simulink model "Block_Leg_PurePursuit"  (R2025b)
settings: Solver=VariableStepAuto  StartTime=0.0  StopTime=80  RelTol=1e-3  AbsTol=1e-3  EnableMultiTasking=on
undefined symbols (not defined in the file): waypoints, X, Y, Z
libraries: sm_lib x58, nesl_utility x34, slpidlib x2, robotalgslib x1, sharedtransform x1
(part 3 of 3)

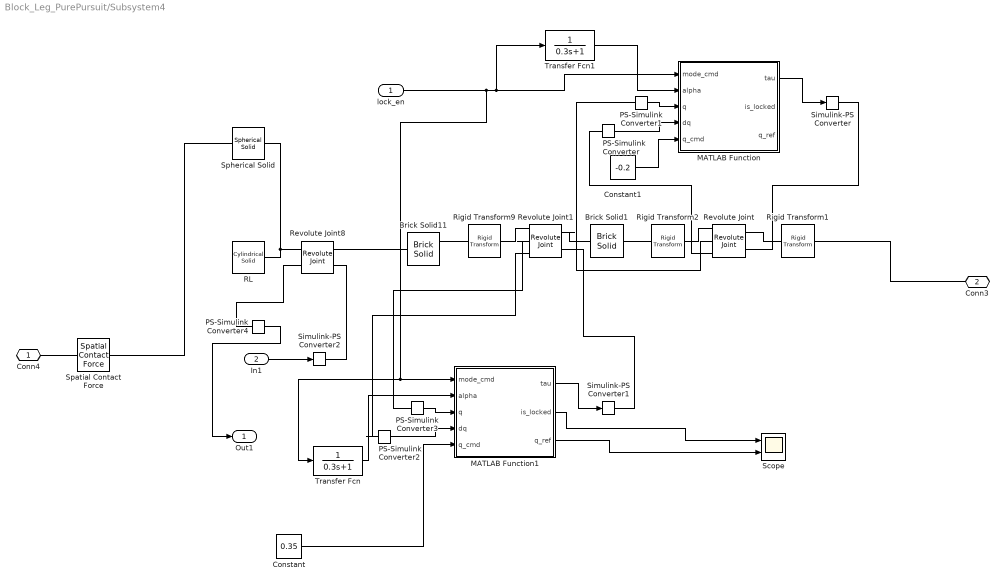
== system Block_Leg_PurePursuit/Subsystem4 ==
  lock_en : Inport
  In1 : Inport  Port=2
  Brick Solid1 : sm_lib/Body Elements/Brick Solid  BrickDimensions=[0.2 0.6 0.2]  BrickDimensionsUnits=m  ExportEntireGeometry=off  InertiaType=CalculateFromGeometry  BasedOnType=Mass  Density=1000  DensityUnits=kg/m^3  Mass=1  MassUnits=kg  CenterOfMass=[0 0 0]  CenterOfMassUnits=m  MomentsOfInertia=[1 1 1]  MomentsOfInertiaUnits=kg*m^2  ProductsOfInertia=[0 0 0]  ProductsOfInertiaUnits=kg*m^2  GraphicType=FromGeometry  MarkerShape=Sphere  MarkerSize=10  GraphicVisPropType=SimpleVisualProperties  GraphicDiffuseColor=[0.6667 1 1]  GraphicOpacity=1  GraphicSpecularColor=[0.5 0.5 0.5 1.0]  GraphicAmbientColor=[0.15 0.15 0.15 1.0]  GraphicEmissiveColor=[0.0 0.0 0.0 1.0]  GraphicShininess=75  DoExposeReferenceFrame=off  SerializedFrames=|
      | <Frames>
      | 
      |   <Frame>
      |     <Id>Frame1</Id>
      |     <Value>
      |       <Name>F1</Name>
      |       <Origin>
      |         <Source>GeometricFeature</Source>
      |         <FeatureName>+x -y +z point</FeatureName>
      |       </Origin>
      |       <PrimaryAxis>
      |         <DefinedDirection>+Z</DefinedDirection>
      |         <Source>ReferenceFrame</Source>
      |         <SourceDirection>+Z</SourceDirection>
      |         <FeatureName></FeatureName>
      |       </PrimaryAxis>
      |       <SecondaryAxis>
      |         <DefinedDirection>+X</DefinedDirection>
      |         <Source>ReferenceFrame</Source>
      |         <SourceDirection>+X</SourceDirection>
      |         <FeatureName></FeatureName>
      |       </SecondaryAxis>
      |     </Value>
      |   </Frame>
      | 
      |   <Frame>
      |     <Id>Frame2</Id>
      |     <Value>
      |       <Name>F2</Name>
      |       <Origin>
      |         <Source>GeometricFeature</Source>
      |         <FeatureName>+y surface</FeatureName>
      |       </Origin>
      |       <PrimaryAxis>
      |         <DefinedDirection>+Z</DefinedDirection>
      |         <Source>ReferenceFrame</Source>
      |         <SourceDirection>+Z</SourceDirection>
      |         <FeatureName></FeatureName>
      |       </PrimaryAxis>
      |       <SecondaryAxis>
      |         <DefinedDirection>+X</DefinedDirection>
      |         <Source>ReferenceFrame</Source>
      |         <SourceDirection>+X</SourceDirection>
      |         <FeatureName></FeatureName>
      |       </SecondaryAxis>
      |     </Value>
      |   </Frame>
      | 
      | </Frames>
  Brick Solid11 : sm_lib/Body Elements/Brick Solid  BrickDimensions=[0.2 1 0.2]  BrickDimensionsUnits=m  ExportEntireGeometry=on  InertiaType=CalculateFromGeometry  BasedOnType=Mass  Density=1000  DensityUnits=kg/m^3  Mass=1  MassUnits=kg  CenterOfMass=[0 0 0]  CenterOfMassUnits=m  MomentsOfInertia=[1 1 1]  MomentsOfInertiaUnits=kg*m^2  ProductsOfInertia=[0 0 0]  ProductsOfInertiaUnits=kg*m^2  GraphicType=FromGeometry  MarkerShape=Sphere  MarkerSize=10  GraphicVisPropType=SimpleVisualProperties  GraphicDiffuseColor=[0.6667 1 1]  GraphicOpacity=1  GraphicSpecularColor=[0.5 0.5 0.5 1.0]  GraphicAmbientColor=[0.15 0.15 0.15 1.0]  GraphicEmissiveColor=[0.0 0.0 0.0 1.0]  GraphicShininess=75  DoExposeReferenceFrame=off  SerializedFrames=|
      | <Frames>
      | 
      |   <Frame>
      |     <Id>Frame1</Id>
      |     <Value>
      |       <Name>F1</Name>
      |       <Origin>
      |         <Source>GeometricFeature</Source>
      |         <FeatureName>+x -y +z point</FeatureName>
      |       </Origin>
      |       <PrimaryAxis>
      |         <DefinedDirection>+Z</DefinedDirection>
      |         <Source>ReferenceFrame</Source>
      |         <SourceDirection>+Z</SourceDirection>
      |         <FeatureName></FeatureName>
      |       </PrimaryAxis>
      |       <SecondaryAxis>
      |         <DefinedDirection>+X</DefinedDirection>
      |         <Source>ReferenceFrame</Source>
      |         <SourceDirection>+X</SourceDirection>
      |         <FeatureName></FeatureName>
      |       </SecondaryAxis>
      |     </Value>
      |   </Frame>
      | 
      |   <Frame>
      |     <Id>Frame2</Id>
      |     <Value>
      |       <Name>F2</Name>
      |       <Origin>
      |         <Source>GeometricFeature</Source>
      |         <FeatureName>+y surface</FeatureName>
      |       </Origin>
      |       <PrimaryAxis>
      |         <DefinedDirection>+Z</DefinedDirection>
      |         <Source>ReferenceFrame</Source>
      |         <SourceDirection>+Z</SourceDirection>
      |         <FeatureName></FeatureName>
      |       </PrimaryAxis>
      |       <SecondaryAxis>
      |         <DefinedDirection>+X</DefinedDirection>
      |         <Source>ReferenceFrame</Source>
      |         <SourceDirection>+X</SourceDirection>
      |         <FeatureName></FeatureName>
      |       </SecondaryAxis>
      |     </Value>
      |   </Frame>
      | 
      | </Frames>
  Constant : Constant  Value=0.35
  Constant1 : Constant  Value=-0.2
  MATLAB Function : MATLAB Function  TreatAsAtomicUnit=on  SystemSampleTime=0.002
  MATLAB Function1 : MATLAB Function  TreatAsAtomicUnit=on  SystemSampleTime=0.002
  PS-Simulink Converter{,1..4} (5 alike) : nesl_utility/PS-Simulink Converter  PhysicalDomain=network_engine_domain  SubClassName=ps_output  LeftPortType=input  RightPortType=output  PseudoPeriodic=off  Frequencies=[]  VectorFormat=inherit  Unit=inherit  AffineConversion=off
  RL : sm_lib/Body Elements/Cylindrical Solid  CylinderRadius=0.5  CylinderRadiusUnits=m  CylinderLength=0.3  CylinderLengthUnits=m  ExportEntireGeometry=on  InertiaType=CalculateFromGeometry  BasedOnType=Mass  Density=1000  DensityUnits=kg/m^3  Mass=0.2  MassUnits=kg  CenterOfMass=[0 0 0]  CenterOfMassUnits=m  MomentsOfInertia=[1 1 1]  MomentsOfInertiaUnits=kg*m^2  ProductsOfInertia=[0 0 0]  ProductsOfInertiaUnits=kg*m^2  GraphicType=FromGeometry  MarkerShape=Sphere  MarkerSize=10  GraphicVisPropType=SimpleVisualProperties  GraphicDiffuseColor=[0.6667 1 1]  GraphicOpacity=1  GraphicSpecularColor=[0.5 0.5 0.5 1.0]  GraphicAmbientColor=[0.15 0.15 0.15 1.0]  GraphicEmissiveColor=[0.0 0.0 0.0 1.0]  GraphicShininess=75  DoExposeReferenceFrame=on  SerializedFrames=<Frames/>
  Revolute Joint : sm_lib/Joints/Revolute Joint  JointMode=Normal  CompositeWrenchDir=FollowerOnBase  CompositeWrenchFrame=BaseFrame  SenseConstraintForce=off  SenseConstraintTorque=off  SenseTotalForce=off  SenseTotalTorque=off  PositionTargetSpecify=off  PositionTargetPriority=High  PositionTargetValue=0  PositionTargetValueUnits=deg  VelocityTargetSpecify=off  VelocityTargetPriority=High  VelocityTargetValue=0  VelocityTargetValueUnits=deg/s  EquilibriumPosition=0  EquilibriumPositionUnits=deg  SpringStiffness=0  SpringStiffnessUnits=N*m/deg  DampingCoefficient=0  DampingCoefficientUnits=N*m/(deg/s)  LowerLimitSpecify=off  LowerLimitBound=-90  LowerLimitBoundUnits=deg  LowerLimitStiffness=1e4  LowerLimitStiffnessUnits=N*m/deg  LowerLimitDamping=10  LowerLimitDampingUnits=N*m/(deg/s)  LowerLimitTransitionRegionWidth=0.1  LowerLimitTransitionRegionWidthUnits=deg  UpperLimitSpecify=off  UpperLimitBound=90  UpperLimitBoundUnits=deg  UpperLimitStiffness=1e4  UpperLimitStiffnessUnits=N*m/deg  UpperLimitDamping=10  UpperLimitDampingUnits=N*m/(deg/s)  UpperLimitTransitionRegionWidth=0.1  UpperLimitTransitionRegionWidthUnits=deg  TorqueActuationMode=InputTorque  MotionActuationMode=ComputedMotion  SensePosition=on  SenseVelocity=on  SenseAcceleration=off  SenseTorqueForce=off  SenseLowerLimitTorqueForce=off  SenseUpperLimitTorqueForce=off
  Revolute Joint1 : sm_lib/Joints/Revolute Joint  JointMode=Normal  CompositeWrenchDir=FollowerOnBase  CompositeWrenchFrame=BaseFrame  SenseConstraintForce=off  SenseConstraintTorque=off  SenseTotalForce=off  SenseTotalTorque=off  PositionTargetSpecify=off  PositionTargetPriority=High  PositionTargetValue=0  PositionTargetValueUnits=deg  VelocityTargetSpecify=off  VelocityTargetPriority=High  VelocityTargetValue=0  VelocityTargetValueUnits=deg/s  EquilibriumPosition=0  EquilibriumPositionUnits=deg  SpringStiffness=0  SpringStiffnessUnits=N*m/deg  DampingCoefficient=0  DampingCoefficientUnits=N*m/(deg/s)  LowerLimitSpecify=off  LowerLimitBound=-90  LowerLimitBoundUnits=deg  LowerLimitStiffness=1e4  LowerLimitStiffnessUnits=N*m/deg  LowerLimitDamping=10  LowerLimitDampingUnits=N*m/(deg/s)  LowerLimitTransitionRegionWidth=0.1  LowerLimitTransitionRegionWidthUnits=deg  UpperLimitSpecify=off  UpperLimitBound=90  UpperLimitBoundUnits=deg  UpperLimitStiffness=1e4  UpperLimitStiffnessUnits=N*m/deg  UpperLimitDamping=10  UpperLimitDampingUnits=N*m/(deg/s)  UpperLimitTransitionRegionWidth=0.1  UpperLimitTransitionRegionWidthUnits=deg  TorqueActuationMode=InputTorque  MotionActuationMode=ComputedMotion  SensePosition=on  SenseVelocity=on  SenseAcceleration=off  SenseTorqueForce=off  SenseLowerLimitTorqueForce=off  SenseUpperLimitTorqueForce=off
  Revolute Joint8 : sm_lib/Joints/Revolute Joint  JointMode=Normal  CompositeWrenchDir=FollowerOnBase  CompositeWrenchFrame=BaseFrame  SenseConstraintForce=off  SenseConstraintTorque=off  SenseTotalForce=off  SenseTotalTorque=off  PositionTargetSpecify=off  PositionTargetPriority=High  PositionTargetValue=0  PositionTargetValueUnits=deg  VelocityTargetSpecify=off  VelocityTargetPriority=High  VelocityTargetValue=0  VelocityTargetValueUnits=deg/s  EquilibriumPosition=0  EquilibriumPositionUnits=deg  SpringStiffness=0  SpringStiffnessUnits=N*m/deg  DampingCoefficient=0  DampingCoefficientUnits=N*m/(deg/s)  LowerLimitSpecify=off  LowerLimitBound=-90  LowerLimitBoundUnits=deg  LowerLimitStiffness=1e4  LowerLimitStiffnessUnits=N*m/deg  LowerLimitDamping=10  LowerLimitDampingUnits=N*m/(deg/s)  LowerLimitTransitionRegionWidth=0.1  LowerLimitTransitionRegionWidthUnits=deg  UpperLimitSpecify=off  UpperLimitBound=90  UpperLimitBoundUnits=deg  UpperLimitStiffness=1e4  UpperLimitStiffnessUnits=N*m/deg  UpperLimitDamping=10  UpperLimitDampingUnits=N*m/(deg/s)  UpperLimitTransitionRegionWidth=0.1  UpperLimitTransitionRegionWidthUnits=deg  TorqueActuationMode=InputTorque  MotionActuationMode=ComputedMotion  SensePosition=off  SenseVelocity=on  SenseAcceleration=off  SenseTorqueForce=off  SenseLowerLimitTorqueForce=off  SenseUpperLimitTorqueForce=off
  Rigid Transform1 : sm_lib/Frames and Transforms/Rigid Transform  RotationMethod=AlignedAxes  FollAlignAxisA=+Z  BaseAlignAxisA=+Y  FollAlignAxisB=+X  BaseAlignAxisB=+X  RotationStandardAxis=+Z  RotationAngle=0  RotationAngleUnits=deg  RotationArbitraryAxis=[0 0 1]  RotationSequenceAxes=FollowerAxes  RotationSequence=XYX  RotationSequenceAngles=[0 0 0]  RotationSequenceAnglesUnits=deg  RotationMatrix=[1 0 0;0 1 0;0 0 1]  Quaternion=[1 0 0 0]  TranslationMethod=None  TranslationCartesianOffset=[0 0 0]  TranslationCartesianOffsetUnits=m  TranslationStandardAxis=+Z  TranslationStandardOffset=0  TranslationStandardOffsetUnits=m  TranslationROffset=0  TranslationROffsetUnits=m  TranslationThetaOffset=0  TranslationThetaOffsetUnits=deg  TranslationZOffset=0  TranslationZOffsetUnits=m
  Rigid Transform2 : sm_lib/Frames and Transforms/Rigid Transform  RotationMethod=RotationSequence  FollAlignAxisA=+X  BaseAlignAxisA=+Y  FollAlignAxisB=+Y  BaseAlignAxisB=+Z  RotationStandardAxis=+Z  RotationAngle=0  RotationAngleUnits=deg  RotationArbitraryAxis=[0 0 1]  RotationSequenceAxes=FollowerAxes  RotationSequence=XYZ  RotationSequenceAngles=[0 0 45]  RotationSequenceAnglesUnits=deg  RotationMatrix=[1 0 0;0 1 0;0 0 1]  Quaternion=[1 0 0 0]  TranslationMethod=None  TranslationCartesianOffset=[0 0 0]  TranslationCartesianOffsetUnits=m  TranslationStandardAxis=+Z  TranslationStandardOffset=0  TranslationStandardOffsetUnits=m  TranslationROffset=0  TranslationROffsetUnits=m  TranslationThetaOffset=0  TranslationThetaOffsetUnits=deg  TranslationZOffset=0  TranslationZOffsetUnits=m
  Rigid Transform9 : sm_lib/Frames and Transforms/Rigid Transform  RotationMethod=RotationSequence  FollAlignAxisA=+X  BaseAlignAxisA=+Y  FollAlignAxisB=+Y  BaseAlignAxisB=+Z  RotationStandardAxis=+Z  RotationAngle=0  RotationAngleUnits=deg  RotationArbitraryAxis=[0 0 1]  RotationSequenceAxes=FollowerAxes  RotationSequence=XYZ  RotationSequenceAngles=[0 0 -75]  RotationSequenceAnglesUnits=deg  RotationMatrix=[1 0 0;0 1 0;0 0 1]  Quaternion=[1 0 0 0]  TranslationMethod=None  TranslationCartesianOffset=[0 0 0]  TranslationCartesianOffsetUnits=m  TranslationStandardAxis=+Z  TranslationStandardOffset=0  TranslationStandardOffsetUnits=m  TranslationROffset=0  TranslationROffsetUnits=m  TranslationThetaOffset=0  TranslationThetaOffsetUnits=deg  TranslationZOffset=0  TranslationZOffsetUnits=m
  Scope : Scope  NumInputPorts=2
      settings: ActiveDisplayYMinimum=-1  ActiveDisplayYMaximum=1
  Simulink-PS Converter : nesl_utility/Simulink-PS Converter  PhysicalDomain=network_engine_domain  SubClassName=ps_input  LeftPortType=input  RightPortType=output  PseudoPeriodic=off  Frequencies=[]  NoiseDistribution=none  NoiseParameters=[]  Unit=1  AffineConversion=off  FilteringAndDerivatives=provide  SimscapeFilterOrder=1  InputFilterTimeConstant=0.001  UdotUserProvided=0
  Simulink-PS Converter1 : nesl_utility/Simulink-PS Converter  PhysicalDomain=network_engine_domain  SubClassName=ps_input  LeftPortType=input  RightPortType=output  PseudoPeriodic=off  Frequencies=[]  NoiseDistribution=none  NoiseParameters=[]  Unit=1  AffineConversion=off  FilteringAndDerivatives=provide  SimscapeFilterOrder=1  InputFilterTimeConstant=0.001  UdotUserProvided=0
  Simulink-PS Converter2 : nesl_utility/Simulink-PS Converter  PhysicalDomain=network_engine_domain  SubClassName=ps_input  LeftPortType=input  RightPortType=output  PseudoPeriodic=off  Frequencies=[]  NoiseDistribution=none  NoiseParameters=[]  Unit=1  AffineConversion=off  FilteringAndDerivatives=provide  SimscapeFilterOrder=1  InputFilterTimeConstant=0.001  UdotUserProvided=0
  Spatial Contact Force : sm_lib/Forces and Torques/Spatial Contact Force  SenseSeparationDistance=off  NormalForceType=SmoothSpringDamper  NormalStiffness=1e6  NormalStiffnessUnits=N/m  NormalDamping=1e3  NormalDampingUnits=N/(m/s)  NormalTransitionRegionWidth=1e-4  NormalTransitionRegionWidthUnits=m  FrictionType=SmoothStickSlip  CoefficientOfStaticFriction=0.9  CoefficientOfDynamicFriction=0.7  FrictionalCriticalVelocity=1e-3  FrictionalCriticalVelocityUnits=m/s  SenseContactSignal=off  SensePenetrationDepth=off  SenseNormalVelocity=off  SenseTangentialVelocity=off  SensingForceTorqueDirection=BaseOnFollower  SensingForceTorqueResolutionFrame=ContactFrame  SenseNormalForce=off  SenseNormalForceMagnitude=off  SenseNormalTorque=off  SenseFrictionalForce=off  SenseFrictionalForceMagnitude=off  SenseFrictionalTorque=off  SenseTotalForce=off  SenseTotalTorque=off  SenseContactBaseRotation=off  SenseContactBaseTranslation=off  SenseContactFollowerRotation=off  SenseContactFollowerTranslation=off  ZeroCrossDetectContactStartAndEnd=off
  Spherical Solid : sm_lib/Body Elements/Spherical Solid  SphereRadius=0.5  SphereRadiusUnits=m  ExportEntireGeometry=on  InertiaType=CalculateFromGeometry  BasedOnType=Mass  Density=1000  DensityUnits=kg/m^3  Mass=0  MassUnits=kg  CenterOfMass=[0 0 0]  CenterOfMassUnits=m  MomentsOfInertia=[1 1 1]  MomentsOfInertiaUnits=kg*m^2  ProductsOfInertia=[0 0 0]  ProductsOfInertiaUnits=kg*m^2  GraphicType=FromGeometry  MarkerShape=Sphere  MarkerSize=10  GraphicVisPropType=SimpleVisualProperties  GraphicDiffuseColor=[1 0 0]  GraphicOpacity=0.2  GraphicSpecularColor=[0.5 0.5 0.5 1.0]  GraphicAmbientColor=[0.15 0.15 0.15 1.0]  GraphicEmissiveColor=[0.0 0.0 0.0 1.0]  GraphicShininess=75  DoExposeReferenceFrame=on  SerializedFrames=<Frames/>
  Transfer Fcn : TransferFcn  Denominator=[0.3 1]
  Transfer Fcn1 : TransferFcn  Denominator=[0.3 1]
  Conn4 : PMIOPort  Side=Left
  Conn3 : PMIOPort  Port=2  Side=Right
  Out1 : Outport
  wires:
  MATLAB Function/1(tau) -> Simulink-PS Converter/1
  PS-Simulink Converter3/1 -> MATLAB Function1/3(q)
  PS-Simulink Converter2/1 -> MATLAB Function1/4(dq)
  PS-Simulink Converter/1 -> MATLAB Function/4(dq)
  PS-Simulink Converter1/1 -> MATLAB Function/3(q)
  MATLAB Function1/1(tau) -> Simulink-PS Converter1/1
  In1/1 -> Simulink-PS Converter2/1
  PS-Simulink Converter4/1 -> Out1/1
  MATLAB Function1/2(is_locked) -> Scope/1
  MATLAB Function1/3(q_ref) -> Scope/2
  Transfer Fcn/1 -> MATLAB Function1/2(alpha)
  Transfer Fcn1/1 -> MATLAB Function/2(alpha)
  lock_en/1 -> Transfer Fcn/1, MATLAB Function1/1(mode_cmd), Transfer Fcn1/1, MATLAB Function/1(mode_cmd)
  Constant/1 -> MATLAB Function1/5(q_cmd)
  Constant1/1 -> MATLAB Function/5(q_cmd)
  connections:
  Revolute Joint/LConn1 -- Rigid Transform1/RConn1
  Simulink-PS Converter1/RConn1 -- Revolute Joint1/LConn2
  Rigid Transform9/LConn1 -- Revolute Joint1/RConn1
  Spherical Solid/LConn1 -- Spatial Contact Force/RConn1
  Brick Solid11/RConn1 -- Revolute Joint8/LConn1
  Revolute Joint1/LConn1 -- Brick Solid1/RConn1
  Revolute Joint8/RConn1 -- RL/RConn1 -- Spherical Solid/RConn1
  Rigid Transform2/LConn1 -- Revolute Joint/RConn1
  Brick Solid11/LConn1 -- Rigid Transform9/RConn1
  Brick Solid1/LConn1 -- Rigid Transform2/RConn1
  Spatial Contact Force/LConn1 -- Conn4/RConn1
  PS-Simulink Converter2/LConn1 -- Revolute Joint1/RConn3
  PS-Simulink Converter/LConn1 -- Revolute Joint/RConn3
  Revolute Joint1/RConn2 -- PS-Simulink Converter3/LConn1
  Simulink-PS Converter/RConn1 -- Revolute Joint/LConn2
  PS-Simulink Converter1/LConn1 -- Revolute Joint/RConn2
  Rigid Transform1/LConn1 -- Conn3/RConn1
  Simulink-PS Converter2/RConn1 -- Revolute Joint8/LConn2
  Revolute Joint8/RConn2 -- PS-Simulink Converter4/LConn1

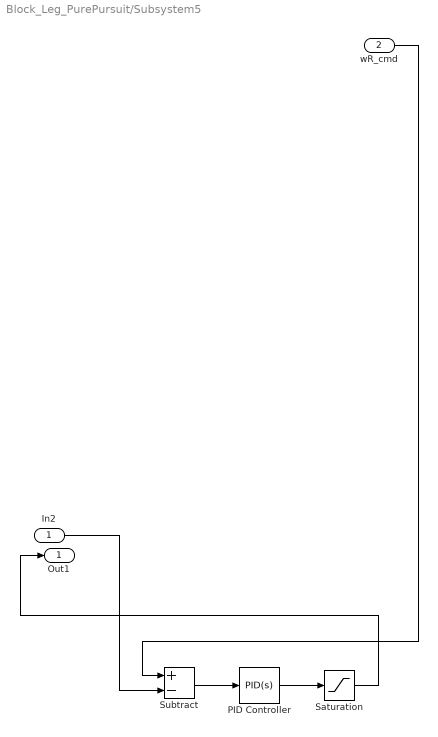
== system Block_Leg_PurePursuit/Subsystem5 ==
  In2 : Inport
  wR_cmd : Inport  Port=2
  PID Controller : slpidlib/PID Controller  Controller=PID  Form=Parallel  TimeDomain=Continuous-time  UseExternalTs=off  SampleTime=-1  IntegratorMethod=Forward Euler  FilterMethod=Forward Euler  ControllerParametersSource=internal  P=5  I=0  UseKiTs=off  D=0  UseExternalDerivativeSource=off  N=100  UseFilter=on  TunerSelectOption=Transfer Function Based (PID Tuner App)  InitialConditionSource=internal  InitialConditionForIntegrator=0  InitialConditionForFilter=0  DifferentiatorICPrevScaledInput=0  ExternalReset=none  TrackingMode=off  Kt=1  LimitOutput=off  SatLimitsSource=internal  UpperSaturationLimit=inf  LowerSaturationLimit=-inf  LinearizeAsGain=on  AntiWindupMode=none  Kb=1  LimitIntegrator=off  UpperIntegratorSaturationLimit=inf  LowerIntegratorSaturationLimit=-inf  POutMin=[]  POutMax=[]  IOutMin=[]  IOutMax=[]  DOutMin=[]  DOutMax=[]  NOutMin=[]  NOutMax=[]  SumOutMin=[]  SumOutMax=[]  SaturationOutMin=[]  SaturationOutMax=[]  PParamMin=[]  PParamMax=[]  IParamMin=[]  IParamMax=[]  DParamMin=[]  DParamMax=[]  NParamMin=[]  NParamMax=[]  KbParamMin=[]  KbParamMax=[]  KtParamMin=[]  KtParamMax=[]  KbOutMin=[]  KbOutMax=[]  KtOutMin=[]  KtOutMax=[]  IntegratorOutMin=[]  IntegratorOutMax=[]  FilterOutMin=[]  FilterOutMax=[]  SumI1OutMin=[]  SumI1OutMax=[]  SumI2OutMin=[]  SumI2OutMax=[]  SumI3OutMin=[]  SumI3OutMax=[]  SumI4OutMin=[]  SumI4OutMax=[]  SumDOutMin=[]  SumDOutMax=[]  DifferentiatorOutMin=[]  DifferentiatorOutMax=[]  FilterDiffOutCoefMin=[]  FilterDiffOutCoefMax=[]  ReciprocalOutMin=[]  ReciprocalOutMax=[]  SumDenOutMin=[]  SumDenOutMax=[]  SumNumOutMin=[]  SumNumOutMax=[]  DivideOutMin=[]  DivideOutMax=[]  UdiffTsProdOutMin=[]  UdiffTsProdOutMax=[]  NTsProdOutMin=[]  NTsProdOutMax=[]  UintegralTsProdOutMin=[]  UintegralTsProdOutMax=[]  UngainTsProdOutMin=[]  UngainTsProdOutMax=[]  ClampingZeroOutDataTypeStr=Inherit: Inherit via back propagation  ClampingZeroOutMin=[]  ClampingZeroOutMax=[]  FilterDenConstantOutDataTypeStr=Inherit: Inherit via back propagation  FilterDenConstantOutMin=[]  FilterDenConstantOutMax=[]  PCopyOutDataTypeStr=Inherit: Inherit via back propagation  PCopyOutMin=[]  PCopyOutMax=[]  NCopyOutDataTypeStr=Inherit: Inherit via back propagation  NCopyOutMin=[]  NCopyOutMax=[]  IntegratorContinuousStateAttributes=''  IntegratorStateMustResolveToSignalObject=off  IntegratorRTWStateStorageClass=Auto  FilterContinuousStateAttributes=''  FilterStateMustResolveToSignalObject=off  FilterRTWStateStorageClass=Auto  ParallelPVariant=InternalParameters  IdealPVariant=Disabled  IVariant=InternalParameters  DVariant=InternalParameters  IntegratorVariant=Continuous  SatVariant=Disabled  AWVariant=Passthrough  PCopyVariant=Disabled  TRVariant=Disabled  FdbkBlocksVariant=Forward  IdealPFdbkVariant=Disabled  SatFdbkVariant=Disabled  DerivativeFilterVariant=ContFilter  NVariant=InternalParameters  NCopyVariant=Disabled  FilterICVariant=InternalICsFilter  IntegratorICVariant=InternalICs  ExternalResetVariant=Disabled  TRSumVariant=Passthrough  SumFdbkVariant=Disabled  SumVariant=Sum_PID  TsampFilterVariant=InternalTs  TsampNgainVariant=Passthrough  TsampIntegralVariant=Disabled_SignalSpec  ExternalSaturationOutDataTypeStr=Inherit: Same as second input  DerivativeSourceVariant=ErrorSignal  PreIntVariant=InternalPreInt
  Saturation : Saturate  UpperLimit=5  LowerLimit=-5
  Subtract : Sum  Inputs=+-
  Out1 : Outport
  wires:
  In2/1 -> Subtract/2
  Subtract/1 -> PID Controller/1
  Saturation/1 -> Out1/1
  PID Controller/1 -> Saturation/1
  wR_cmd/1 -> Subtract/1

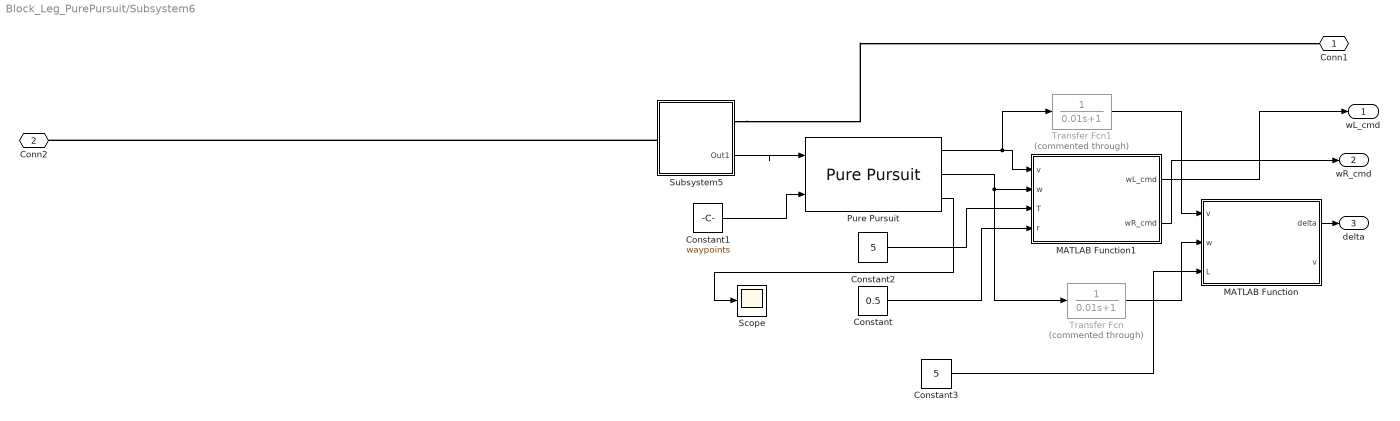
== system Block_Leg_PurePursuit/Subsystem6 ==
  Constant : Constant  Value=0.5
  Constant1 : Constant  Value=waypoints
  Constant2 : Constant  Value=5
  Constant3 : Constant  Value=5
  MATLAB Function : MATLAB Function  TreatAsAtomicUnit=on
  MATLAB Function1 : MATLAB Function  TreatAsAtomicUnit=on
  Pure Pursuit : robotalgslib/Pure Pursuit  DesiredLinearVelocityPort=off  DesiredLinearVelocity=3  MaxAngularVelocity=2  LookaheadDistancePort=off  LookaheadDistance=4  TargetDirPort=on  SimulateUsing=Code generation
      settings: LibrarySourceBlock=navlib/Control Algorithms/Pure Pursuit
  Scope : Scope
      settings: ActiveDisplayYMinimum=-4.8040636325719674  ActiveDisplayYMaximum=3.5962705540777251
  Subsystem5 : Subsystem
      settings: PortSchema="{\"entries\":[{\"content\":{\"sides\":[{\"content\":{\"connectorIds\":[\"LConn1\"]},\"type\":\"ConnectorPlacement.EquallySpacedRectSide\",\"uuid\":\"ddf93349-53d1-49a0-944e-d0734f46f29a\"},{\"content\":{\"connectorIds\":[\"RConn1\",\"Out1\"],\"side\":\"RIGHT\"},\"type\":\"ConnectorPlacement.EquallySpacedRectSide\",\"uuid\":\"41423d35-5168-4258-b195-077866701bba\"},{\"content\":{\"side\":\"TOP\"},\"type\":\"ConnectorPlacement.EquallySpacedRectSide\",\"uuid\":\"a64c51dc-c679-4f29-97b2-168705ea0e49\"}]},\"type\":\"ConnectorPlacement.EquallySpacedConnector\",\"uuid\":\"ed4aabc3-31ac-4b26-a964-31268bbe4985\"}],\"packageUris\":[\"http://schema.mathworks.com/mf0/Connector/R2020b\"],\"version\":\"1.0\"}"
  Transfer Fcn : TransferFcn  Commented=through  Denominator=[0.01 1]
  Transfer Fcn1 : TransferFcn  Commented=through  Denominator=[0.01 1]
  Conn1 : PMIOPort  Side=Right
  Conn2 : PMIOPort  Port=2  Side=Left
  wL_cmd : Outport
  wR_cmd : Outport  Port=2
  delta : Outport  Port=3
  wires:
  Pure Pursuit/2 -> Transfer Fcn/1, MATLAB Function1/2(w)
  Transfer Fcn1/1 -> MATLAB Function/1("v ")
  Transfer Fcn/1 -> MATLAB Function/2(w)
  Constant1/1 -> Pure Pursuit/2
  MATLAB Function/1(delta) -> delta/1
  Constant/1 -> MATLAB Function1/4(r)
  Constant2/1 -> MATLAB Function1/3(T)
  Constant3/1 -> MATLAB Function/3(L)
  MATLAB Function1/2(wR_cmd) -> wR_cmd/1
  MATLAB Function1/1(wL_cmd) -> wL_cmd/1
  Pure Pursuit/1 -> Transfer Fcn1/1, MATLAB Function1/1(v)
  Pure Pursuit/3 -> Scope/1
  Subsystem5/1(Out1) -> Pure Pursuit/1
  connections:
  Subsystem5/RConn1 -- Conn1/RConn1
  Subsystem5/LConn1 -- Conn2/RConn1

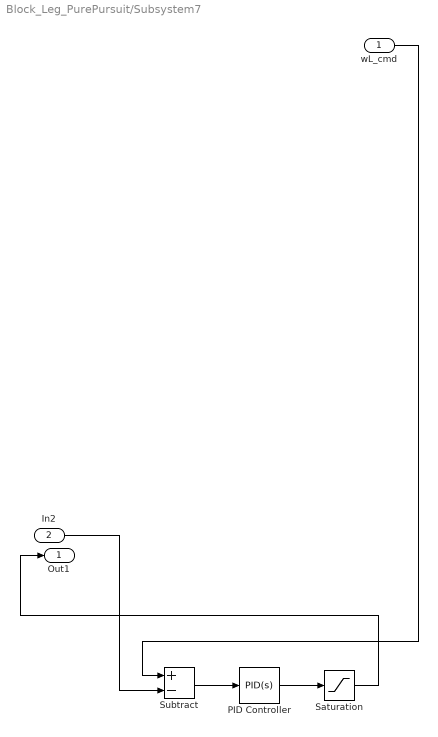
== system Block_Leg_PurePursuit/Subsystem7 ==
  wL_cmd : Inport
  In2 : Inport  Port=2
  PID Controller : slpidlib/PID Controller  Controller=PID  Form=Parallel  TimeDomain=Continuous-time  UseExternalTs=off  SampleTime=-1  IntegratorMethod=Forward Euler  FilterMethod=Forward Euler  ControllerParametersSource=internal  P=5  I=0  UseKiTs=off  D=0  UseExternalDerivativeSource=off  N=100  UseFilter=on  TunerSelectOption=Transfer Function Based (PID Tuner App)  InitialConditionSource=internal  InitialConditionForIntegrator=0  InitialConditionForFilter=0  DifferentiatorICPrevScaledInput=0  ExternalReset=none  TrackingMode=off  Kt=1  LimitOutput=off  SatLimitsSource=internal  UpperSaturationLimit=inf  LowerSaturationLimit=-inf  LinearizeAsGain=on  AntiWindupMode=none  Kb=1  LimitIntegrator=off  UpperIntegratorSaturationLimit=inf  LowerIntegratorSaturationLimit=-inf  POutMin=[]  POutMax=[]  IOutMin=[]  IOutMax=[]  DOutMin=[]  DOutMax=[]  NOutMin=[]  NOutMax=[]  SumOutMin=[]  SumOutMax=[]  SaturationOutMin=[]  SaturationOutMax=[]  PParamMin=[]  PParamMax=[]  IParamMin=[]  IParamMax=[]  DParamMin=[]  DParamMax=[]  NParamMin=[]  NParamMax=[]  KbParamMin=[]  KbParamMax=[]  KtParamMin=[]  KtParamMax=[]  KbOutMin=[]  KbOutMax=[]  KtOutMin=[]  KtOutMax=[]  IntegratorOutMin=[]  IntegratorOutMax=[]  FilterOutMin=[]  FilterOutMax=[]  SumI1OutMin=[]  SumI1OutMax=[]  SumI2OutMin=[]  SumI2OutMax=[]  SumI3OutMin=[]  SumI3OutMax=[]  SumI4OutMin=[]  SumI4OutMax=[]  SumDOutMin=[]  SumDOutMax=[]  DifferentiatorOutMin=[]  DifferentiatorOutMax=[]  FilterDiffOutCoefMin=[]  FilterDiffOutCoefMax=[]  ReciprocalOutMin=[]  ReciprocalOutMax=[]  SumDenOutMin=[]  SumDenOutMax=[]  SumNumOutMin=[]  SumNumOutMax=[]  DivideOutMin=[]  DivideOutMax=[]  UdiffTsProdOutMin=[]  UdiffTsProdOutMax=[]  NTsProdOutMin=[]  NTsProdOutMax=[]  UintegralTsProdOutMin=[]  UintegralTsProdOutMax=[]  UngainTsProdOutMin=[]  UngainTsProdOutMax=[]  ClampingZeroOutDataTypeStr=Inherit: Inherit via back propagation  ClampingZeroOutMin=[]  ClampingZeroOutMax=[]  FilterDenConstantOutDataTypeStr=Inherit: Inherit via back propagation  FilterDenConstantOutMin=[]  FilterDenConstantOutMax=[]  PCopyOutDataTypeStr=Inherit: Inherit via back propagation  PCopyOutMin=[]  PCopyOutMax=[]  NCopyOutDataTypeStr=Inherit: Inherit via back propagation  NCopyOutMin=[]  NCopyOutMax=[]  IntegratorContinuousStateAttributes=''  IntegratorStateMustResolveToSignalObject=off  IntegratorRTWStateStorageClass=Auto  FilterContinuousStateAttributes=''  FilterStateMustResolveToSignalObject=off  FilterRTWStateStorageClass=Auto  ParallelPVariant=InternalParameters  IdealPVariant=Disabled  IVariant=InternalParameters  DVariant=InternalParameters  IntegratorVariant=Continuous  SatVariant=Disabled  AWVariant=Passthrough  PCopyVariant=Disabled  TRVariant=Disabled  FdbkBlocksVariant=Forward  IdealPFdbkVariant=Disabled  SatFdbkVariant=Disabled  DerivativeFilterVariant=ContFilter  NVariant=InternalParameters  NCopyVariant=Disabled  FilterICVariant=InternalICsFilter  IntegratorICVariant=InternalICs  ExternalResetVariant=Disabled  TRSumVariant=Passthrough  SumFdbkVariant=Disabled  SumVariant=Sum_PID  TsampFilterVariant=InternalTs  TsampNgainVariant=Passthrough  TsampIntegralVariant=Disabled_SignalSpec  ExternalSaturationOutDataTypeStr=Inherit: Same as second input  DerivativeSourceVariant=ErrorSignal  PreIntVariant=InternalPreInt
  Saturation : Saturate  UpperLimit=5  LowerLimit=-5
  Subtract : Sum  Inputs=+-
  Out1 : Outport
  wires:
  In2/1 -> Subtract/2
  Subtract/1 -> PID Controller/1
  Saturation/1 -> Out1/1
  PID Controller/1 -> Saturation/1
  wL_cmd/1 -> Subtract/1

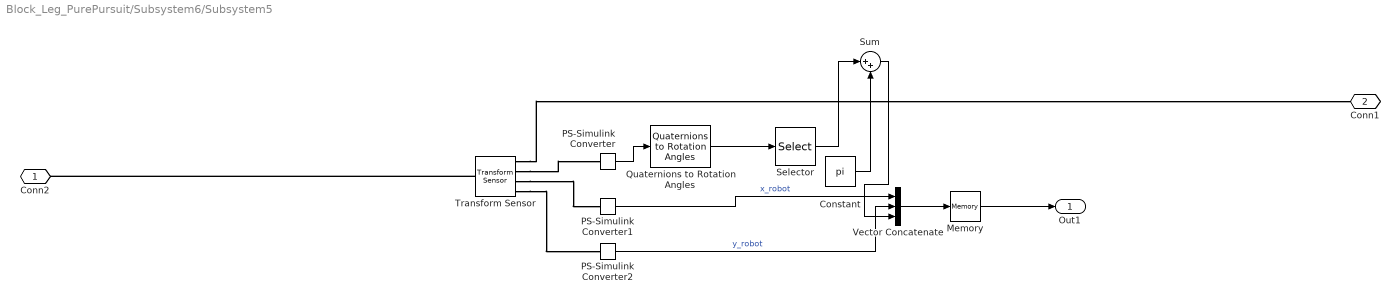
== system Block_Leg_PurePursuit/Subsystem6/Subsystem5 ==
  Constant : Constant  Value=pi
  Memory : Memory
  PS-Simulink Converter : nesl_utility/PS-Simulink Converter  PhysicalDomain=network_engine_domain  SubClassName=ps_output  LeftPortType=input  RightPortType=output  PseudoPeriodic=off  Frequencies=[]  VectorFormat=inherit  Unit=inherit  AffineConversion=off
  PS-Simulink Converter1 : nesl_utility/PS-Simulink Converter  PhysicalDomain=network_engine_domain  SubClassName=ps_output  LeftPortType=input  RightPortType=output  PseudoPeriodic=off  Frequencies=[]  VectorFormat=inherit  Unit=inherit  AffineConversion=off
  PS-Simulink Converter2 : nesl_utility/PS-Simulink Converter  PhysicalDomain=network_engine_domain  SubClassName=ps_output  LeftPortType=input  RightPortType=output  PseudoPeriodic=off  Frequencies=[]  VectorFormat=inherit  Unit=inherit  AffineConversion=off
  Quaternions to Rotation Angles : sharedtransform/Quaternions to Rotation Angles  rotationOrder=ZYX  aMode=aMode
  Selector : Selector  InputPortWidth=3  IndexOptions=Index vector (dialog)  Indices=[1]  OutputSizes=1
  Sum : Sum  Inputs=|++
  Transform Sensor : sm_lib/Frames and Transforms/Transform Sensor  MeasurementFrame=World  RotationSequence=XYX  SenseAngle=off  SenseAxis=off  SenseQ=on  SenseR=off  SenseRotationSequence=off  SenseOmegaX=off  SenseOmegaY=off  SenseOmegaZ=off  SenseOmega=off  SenseQDot=off  SenseRDot=off  SenseRotationSequenceDot=off  SenseAlphaX=off  SenseAlphaY=off  SenseAlphaZ=off  SenseAlpha=off  SenseQDDot=off  SenseRDDot=off  SenseX=on  SenseY=on  SenseZ=off  SenseXYZ=off  SenseRad=off  SenseAzim=off  SenseDist=off  SenseInc=off  SenseXDot=off  SenseYDot=off  SenseZDot=off  SenseXYZDot=off  SenseRadDot=off  SenseAzimDot=off  SenseDistDot=off  SenseIncDot=off  SenseXDDot=off  SenseYDDot=off  SenseZDDot=off  SenseXYZDDot=off  SenseRadDDot=off  SenseAzimDDot=off  SenseDistDDot=off  SenseIncDDot=off
  Vector Concatenate : Concatenate  NumInputs=3
  Conn2 : PMIOPort  Side=Left
  Conn1 : PMIOPort  Port=2  Side=Right
  Out1 : Outport
  wires:
  Quaternions to Rotation Angles/1 -> Selector/1
  PS-Simulink Converter/1 -> Quaternions to Rotation Angles/1
  Vector Concatenate/1 -> Memory/1
  Memory/1 -> Out1/1
  PS-Simulink Converter1/1 -> Vector Concatenate/1  "x_robot"
  PS-Simulink Converter2/1 -> Vector Concatenate/2  "y_robot"
  Selector/1 -> Sum/1
  Constant/1 -> Sum/2
  Sum/1 -> Vector Concatenate/3
  connections:
  Transform Sensor/LConn1 -- Conn2/RConn1
  Transform Sensor/RConn4 -- PS-Simulink Converter2/LConn1
  Transform Sensor/RConn2 -- PS-Simulink Converter/LConn1
  Transform Sensor/RConn3 -- PS-Simulink Converter1/LConn1
  Transform Sensor/RConn1 -- Conn1/RConn1

== matlab function Block_Leg_PurePursuit/Subsystem4/MATLAB Function1 ==
  data: mode_cmd input; alpha input; tau output; q input; dq input; q_cmd input; is_locked output; q_ref output
function [tau, is_locked, q_ref] = LockJointPD(mode_cmd, alpha, q, dq, q_cmd)
%#codegen
% mode_cmd: 0=走路(跟踪q_cmd), 1=轮式(锁当前角)
% alpha   : [0,1] 平滑因子(TransferFcn输出)，0=全走路, 1=全锁腿
% q,dq    : 关节角/角速度
% q_cmd   : 走路/站立目标角(弧度)

Kp = 1200.0;   % 起步值，按关节调
Kd =   20.0;
tau_lim = 300.0;

m = uint8(mode_cmd ~= 0);     % 统一成 uint8(0/1)
a = double(alpha);

persistent q_hold last_mode
if isempty(q_hold),    q_hold    = q;        end   % double
if isempty(last_mode), last_mode = uint8(0); end   % uint8

% 上升沿: 0->1 时锁存当前角
if (last_mode == uint8(0)) && (m ~= uint8(0))
    q_hold = q;
end
last_mode = m;

% 参考角: 在“锁定角”和“目标角”间插值
q_ref  = a*q_hold + (1-a)*q_cmd;
dq_ref = 0.0;

% PD
tau = Kp*(q_ref - q) + Kd*(dq_ref - dq);

% 限幅
tau = max(min(tau, tau_lim), -tau_lim);

% 调试标志：是否处于锁腿主导
is_locked = (a > 0.5);     % 也可输出 m==1
end

== matlab function Block_Leg_PurePursuit/Subsystem6/MATLAB Function1 ==
  data: v input; wL_cmd output; w input; T input; r input; wR_cmd output
function [wL_cmd, wR_cmd] = wheelSpeedCmd(v, w, T, r)
% v: 线速度 [m/s]
% w: 航向角速度 [rad/s]
% T: 后轮距 [m]
% r: 车轮半径 [m]

vL = v - 0.5*T*w;
vR = v + 0.5*T*w;

wL_cmd = vL / r;
wR_cmd = vR / r;
end

== matlab function Block_Leg_PurePursuit/Subsystem6/MATLAB Function ==
  data: v input; delta output; w input; L input; v output
function [delta, v] = Diff2Ackermann(v, w, L)
% input: 
%   v - Linear velocity (m/s)
%   w - Angular velocity (rad/s)
%   L -  (m)
%
% output:
%   delta - front wheel rotation angel (rad)
%   v     -  velocity(m/s)
if abs(v) < 1e-3
    delta = 0;
else
    delta = atan(L * w / v);   % pure pursuit function
end

== matlab function Block_Leg_PurePursuit/Subsystem1/MATLAB Function1 ==
  data: mode_cmd input; alpha input; tau output; q input; dq input; q_cmd input; is_locked output; q_ref output
function [tau, is_locked, q_ref] = LockJointPD(mode_cmd, alpha, q, dq, q_cmd)
%#codegen
% mode_cmd: 0=走路(跟踪q_cmd), 1=轮式(锁当前角)
% alpha   : [0,1] 平滑因子(TransferFcn输出)，0=全走路, 1=全锁腿
% q,dq    : 关节角/角速度
% q_cmd   : 走路/站立目标角(弧度)

Kp = 1200.0;   % 起步值，按关节调
Kd =   20.0;
tau_lim = 300.0;

m = uint8(mode_cmd ~= 0);     % 统一成 uint8(0/1)
a = double(alpha);

persistent q_hold last_mode
if isempty(q_hold),    q_hold    = q;        end   % double
if isempty(last_mode), last_mode = uint8(0); end   % uint8

% 上升沿: 0->1 时锁存当前角
if (last_mode == uint8(0)) && (m ~= uint8(0))
    q_hold = q;
end
last_mode = m;

% 参考角: 在“锁定角”和“目标角”间插值
q_ref  = a*q_hold + (1-a)*q_cmd;
dq_ref = 0.0;

% PD
tau = Kp*(q_ref - q) + Kd*(dq_ref - dq);

% 限幅
tau = max(min(tau, tau_lim), -tau_lim);

% 调试标志：是否处于锁腿主导
is_locked = (a > 0.5);     % 也可输出 m==1
end

== matlab function Block_Leg_PurePursuit/Subsystem1/MATLAB Function ==
  data: mode_cmd input; alpha input; tau output; q input; dq input; q_cmd input; is_locked output; q_ref output
function [tau, is_locked, q_ref] = LockJointPD(mode_cmd, alpha, q, dq, q_cmd)
%#codegen
% mode_cmd: 0=Walk(folloew q_cmd), 1=Wheel(lock the present angle )
% alpha   : [0,1] flatten faktor(TransferFcnoutput)，0=walk, 1=leg locked
% q,dq    : joint angle/angular velocity
% q_cmd   : walking/standing angle(rad)

Kp = 1200.0;   % start value
Kd =   20.0;
tau_lim = 300.0;

m = uint8(mode_cmd ~= 0);     % uint8(0/1)
a = double(alpha);

persistent q_hold last_mode
if isempty(q_hold),    q_hold    = q;        end   % double
if isempty(last_mode), last_mode = uint8(0); end   % uint8

% step: 0->1 
if (last_mode == uint8(0)) && (m ~= uint8(0))
    q_hold = q;
end
last_mode = m;

% reference angle
q_ref  = a*q_hold + (1-a)*q_cmd;
dq_ref = 0.0;

% PD
tau = Kp*(q_ref - q) + Kd*(dq_ref - dq);

% 
tau = max(min(tau, tau_lim), -tau_lim);

% 
is_locked = (a > 0.5);     % 
end

== matlab function Block_Leg_PurePursuit/Subsystem2/MATLAB Function ==
  data: mode_cmd input; alpha input; tau output; q input; dq input; q_cmd input; is_locked output; q_ref output
function [tau, is_locked, q_ref] = LockJointPD(mode_cmd, alpha, q, dq, q_cmd)
%#codegen
% mode_cmd: 0=走路(跟踪q_cmd), 1=轮式(锁当前角)
% alpha   : [0,1] 平滑因子(TransferFcn输出)，0=全走路, 1=全锁腿
% q,dq    : 关节角/角速度
% q_cmd   : 走路/站立目标角(弧度)

Kp = 1200.0;   % 起步值，按关节调
Kd =   20.0;
tau_lim = 300.0;

m = uint8(mode_cmd ~= 0);     % 统一成 uint8(0/1)
a = double(alpha);

persistent q_hold last_mode
if isempty(q_hold),    q_hold    = q;        end   % double
if isempty(last_mode), last_mode = uint8(0); end   % uint8

% 上升沿: 0->1 时锁存当前角
if (last_mode == uint8(0)) && (m ~= uint8(0))
    q_hold = q;
end
last_mode = m;

% 参考角: 在“锁定角”和“目标角”间插值
q_ref  = a*q_hold + (1-a)*q_cmd;
dq_ref = 0.0;

% PD
tau = Kp*(q_ref - q) + Kd*(dq_ref - dq);

% 限幅
tau = max(min(tau, tau_lim), -tau_lim);

% 调试标志：是否处于锁腿主导
is_locked = (a > 0.5);     % 也可输出 m==1
end

== matlab function Block_Leg_PurePursuit/Subsystem2/MATLAB Function1 ==
  data: mode_cmd input; alpha input; tau output; q input; dq input; q_cmd input; is_locked output; q_ref output
function [tau, is_locked, q_ref] = LockJointPD(mode_cmd, alpha, q, dq, q_cmd)
%#codegen
% mode_cmd: 0=走路(跟踪q_cmd), 1=轮式(锁当前角)
% alpha   : [0,1] 平滑因子(TransferFcn输出)，0=全走路, 1=全锁腿
% q,dq    : 关节角/角速度
% q_cmd   : 走路/站立目标角(弧度)

Kp = 1200.0;   % 起步值，按关节调
Kd =   20.0;
tau_lim = 300.0;

m = uint8(mode_cmd ~= 0);     % 统一成 uint8(0/1)
a = double(alpha);

persistent q_hold last_mode
if isempty(q_hold),    q_hold    = q;        end   % double
if isempty(last_mode), last_mode = uint8(0); end   % uint8

% 上升沿: 0->1 时锁存当前角
if (last_mode == uint8(0)) && (m ~= uint8(0))
    q_hold = q;
end
last_mode = m;

% 参考角: 在“锁定角”和“目标角”间插值
q_ref  = a*q_hold + (1-a)*q_cmd;
dq_ref = 0.0;

% PD
tau = Kp*(q_ref - q) + Kd*(dq_ref - dq);

% 限幅
tau = max(min(tau, tau_lim), -tau_lim);

% 调试标志：是否处于锁腿主导
is_locked = (a > 0.5);     % 也可输出 m==1
end

== matlab function Block_Leg_PurePursuit/Subsystem3/MATLAB Function ==
  data: mode_cmd input; alpha input; tau output; q input; dq input; q_cmd input; is_locked output; q_ref output
function [tau, is_locked, q_ref] = LockJointPD(mode_cmd, alpha, q, dq, q_cmd)
%#codegen
% mode_cmd: 0=走路(跟踪q_cmd), 1=轮式(锁当前角)
% alpha   : [0,1] 平滑因子(TransferFcn输出)，0=全走路, 1=全锁腿
% q,dq    : 关节角/角速度
% q_cmd   : 走路/站立目标角(弧度)

Kp = 1200.0;   % 起步值，按关节调
Kd =   20.0;
tau_lim = 300.0;

m = uint8(mode_cmd ~= 0);     % 统一成 uint8(0/1)
a = double(alpha);

persistent q_hold last_mode
if isempty(q_hold),    q_hold    = q;        end   % double
if isempty(last_mode), last_mode = uint8(0); end   % uint8

% 上升沿: 0->1 时锁存当前角
if (last_mode == uint8(0)) && (m ~= uint8(0))
    q_hold = q;
end
last_mode = m;

% 参考角: 在“锁定角”和“目标角”间插值
q_ref  = a*q_hold + (1-a)*q_cmd;
dq_ref = 0.0;

% PD
tau = Kp*(q_ref - q) + Kd*(dq_ref - dq);

% 限幅
tau = max(min(tau, tau_lim), -tau_lim);

% 调试标志：是否处于锁腿主导
is_locked = (a > 0.5);     % 也可输出 m==1
end

== matlab function Block_Leg_PurePursuit/Subsystem3/MATLAB Function1 ==
  data: mode_cmd input; alpha input; tau output; q input; dq input; q_cmd input; is_locked output; q_ref output
function [tau, is_locked, q_ref] = LockJointPD(mode_cmd, alpha, q, dq, q_cmd)
%#codegen
% mode_cmd: 0=走路(跟踪q_cmd), 1=轮式(锁当前角)
% alpha   : [0,1] 平滑因子(TransferFcn输出)，0=全走路, 1=全锁腿
% q,dq    : 关节角/角速度
% q_cmd   : 走路/站立目标角(弧度)

Kp = 1200.0;   % 起步值，按关节调
Kd =   20.0;
tau_lim = 300.0;

m = uint8(mode_cmd ~= 0);     % 统一成 uint8(0/1)
a = double(alpha);

persistent q_hold last_mode
if isempty(q_hold),    q_hold    = q;        end   % double
if isempty(last_mode), last_mode = uint8(0); end   % uint8

% 上升沿: 0->1 时锁存当前角
if (last_mode == uint8(0)) && (m ~= uint8(0))
    q_hold = q;
end
last_mode = m;

% 参考角: 在“锁定角”和“目标角”间插值
q_ref  = a*q_hold + (1-a)*q_cmd;
dq_ref = 0.0;

% PD
tau = Kp*(q_ref - q) + Kd*(dq_ref - dq);

% 限幅
tau = max(min(tau, tau_lim), -tau_lim);

% 调试标志：是否处于锁腿主导
is_locked = (a > 0.5);     % 也可输出 m==1
end

== matlab function Block_Leg_PurePursuit/Subsystem4/MATLAB Function ==
  data: mode_cmd input; alpha input; tau output; q input; dq input; q_cmd input; is_locked output; q_ref output
function [tau, is_locked, q_ref] = LockJointPD(mode_cmd, alpha, q, dq, q_cmd)
%#codegen
% mode_cmd: 0=走路(跟踪q_cmd), 1=轮式(锁当前角)
% alpha   : [0,1] 平滑因子(TransferFcn输出)，0=全走路, 1=全锁腿
% q,dq    : 关节角/角速度
% q_cmd   : 走路/站立目标角(弧度)

Kp = 1200.0;   % 起步值，按关节调
Kd =   20.0;
tau_lim = 300.0;

m = uint8(mode_cmd ~= 0);     % 统一成 uint8(0/1)
a = double(alpha);

persistent q_hold last_mode
if isempty(q_hold),    q_hold    = q;        end   % double
if isempty(last_mode), last_mode = uint8(0); end   % uint8

% 上升沿: 0->1 时锁存当前角
if (last_mode == uint8(0)) && (m ~= uint8(0))
    q_hold = q;
end
last_mode = m;

% 参考角: 在“锁定角”和“目标角”间插值
q_ref  = a*q_hold + (1-a)*q_cmd;
dq_ref = 0.0;

% PD
tau = Kp*(q_ref - q) + Kd*(dq_ref - dq);

% 限幅
tau = max(min(tau, tau_lim), -tau_lim);

% 调试标志：是否处于锁腿主导
is_locked = (a > 0.5);     % 也可输出 m==1
end
